simulink model "autonomous_vehicle"  (R2026a)
settings: Solver=VariableStepAuto  StopTime=2
values from neighbouring files (symbols this model uses):
  b = 2e-5    (= 2e-05)    [init_parameters.m]
  J = 2e-5    (= 2e-05)    [init_parameters.m]
  Ke = 0.02    [init_parameters.m]
  Kt = 0.02    [init_parameters.m]
  Ktheta = 2.0    (= 2)    [init_parameters.m]
  Ky = 1.0    (= 1)    [init_parameters.m]
  L = 2e-3    (= 0.002)    [init_parameters.m]
  R = 4    [init_parameters.m]
  theta0 = 0    [init_parameters.m]
  Vbase = 3.5    [init_parameters.m]
  Vmax = 6    [init_parameters.m]
  wheelDistance = 0.14    [init_parameters.m]
  wheelRadius = 0.0325    [init_parameters.m]
  x0 = 0    [init_parameters.m]
  y0 = 0.10    (= 0.1)    [init_parameters.m]
settings Model: Creator=aliad  LastModifiedBy=aliad

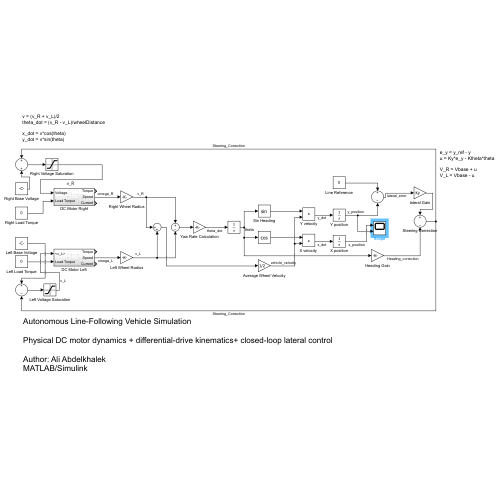
[thumbnail: Simulink's stored preview of the top-level diagram]
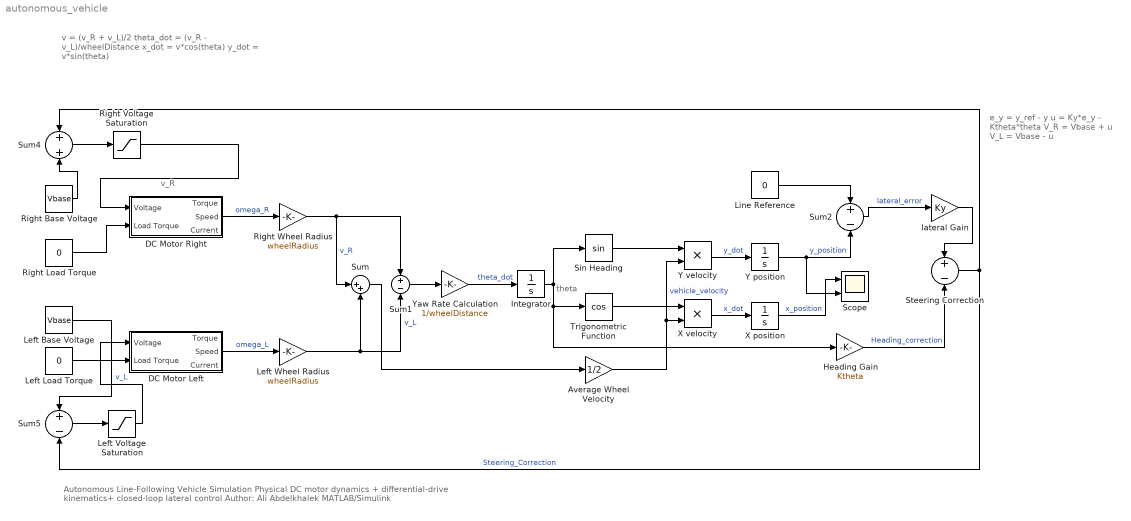
== system autonomous_vehicle ==
  note: v = (v_R + v_L)/2
      | theta_dot = (v_R - v_L)/wheelDistance
      |
      | x_dot = v*cos(theta)
      | y_dot = v*sin(theta)
  note: e_y = y_ref - y
      | u = Ky*e_y - Ktheta*theta
      |
      | V_R = Vbase + u
      | V_L = Vbase - u
  note: Autonomous Line-Following Vehicle Simulation
      |
      | Physical DC motor dynamics + differential-drive kinematics+ closed-loop lateral control
      |
      | Author: Ali Abdelkhalek
      | MATLAB/Simulink
  note: theta
  note: v_R
  "Average Wheel Velocity " : Gain  Gain=1/2
  DC Motor Left : Subsystem
  DC Motor Right : Subsystem
  Heading Gain : Gain  Gain=Ktheta
  Integrator : Integrator  InitialCondition=theta0
  Left Base Voltage : Constant  Value=Vbase
  Left Load Torque : Constant  Value=0
  Left Voltage Saturation : Saturate  UpperLimit=Vmax  LowerLimit=0
  Left Wheel Radius : Gain  Gain=wheelRadius
  Line Reference : Constant  Value=0
  Right Base Voltage : Constant  Value=Vbase
  Right Load Torque : Constant  Value=0
  Right Voltage Saturation : Saturate  UpperLimit=Vmax  LowerLimit=0
  Right Wheel Radius : Gain  Gain=wheelRadius
  Scope : Scope  NumInputPorts=2
      settings: ActiveDisplayYMinimum=-2.1385150832393238  ActiveDisplayYMaximum=5.3992745742207013
  Sin Heading : Trigonometry
  Steering Correction : Sum  Inputs=+-
  Sum : Sum  Inputs=|++
  Sum1 : Sum  Inputs=+-
  Sum2 : Sum  Inputs=+-
  Sum4 : Sum
  Sum5 : Sum  Inputs=+-
  Trigonometric Function : Trigonometry  Operator=cos
  X position : Integrator  InitialCondition=x0
  "X velocity " : Product
  Y position : Integrator  InitialCondition=y0
  Y velocity : Product
  Yaw Rate Calculation : Gain  Gain=1/wheelDistance
  lateral Gain : Gain  Gain=Ky
  wires:
  Left Load Torque/1 -> DC Motor Left/2(Load Torque)
  DC Motor Left/2(Speed) -> Left Wheel Radius/1  "omega_L"
  DC Motor Right/2(Speed) -> Right Wheel Radius/1  "omega_R"
  Right Load Torque/1 -> DC Motor Right/2(Load Torque)
  Sum/1 -> "Average Wheel Velocity "/1
  Left Wheel Radius/1 -> Sum1/2, Sum/2  "v_L"
  Right Wheel Radius/1 -> Sum1/1, Sum/1  "v_R"
  Sum1/1 -> Yaw Rate Calculation/1
  Yaw Rate Calculation/1 -> Integrator/1  "theta_dot"
  Integrator/1 -> Sin Heading/1, Heading Gain/1, Trigonometric Function/1
  Trigonometric Function/1 -> "X velocity "/1
  "Average Wheel Velocity "/1 -> Y velocity/2, "X velocity "/2  "vehicle_velocity"
  "X velocity "/1 -> X position/1  "x_dot"
  Sin Heading/1 -> Y velocity/1
  Y velocity/1 -> Y position/1  "y_dot"
  Y position/1 -> Scope/2, Sum2/2  "y_position"
  Line Reference/1 -> Sum2/1
  Sum2/1 -> lateral Gain/1  "lateral_error"
  lateral Gain/1 -> Steering Correction/1
  Heading Gain/1 -> Steering Correction/2  "Heading_correction"
  Steering Correction/1 -> Sum5/2, Sum4/1  "Steering_Correction"
  Right Base Voltage/1 -> Sum4/2
  Left Base Voltage/1 -> Sum5/1
  Sum4/1 -> Right Voltage Saturation/1
  Right Voltage Saturation/1 -> DC Motor Right/1(Voltage)
  Sum5/1 -> Left Voltage Saturation/1
  Left Voltage Saturation/1 -> DC Motor Left/1(Voltage)  "v_L"
  X position/1 -> Scope/1  "x_position"

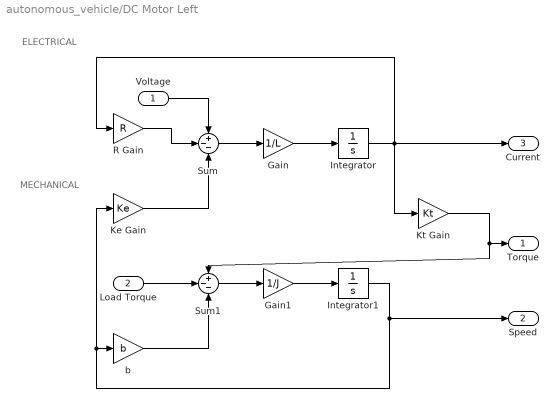
== system autonomous_vehicle/DC Motor Left ==
  note: ELECTRICAL
  note: MECHANICAL
  Voltage : Inport
  Load Torque : Inport  Port=2
  Gain : Gain  Gain=1/L
  Gain1 : Gain  Gain=1/J
  Integrator : Integrator
  Integrator1 : Integrator
  Ke Gain : Gain  Gain=Ke
  Kt Gain : Gain  Gain=Kt
  R Gain : Gain  Gain=R
  Sum : Sum  Inputs=+--
  Sum1 : Sum  Inputs=+--
  b : Gain  Gain=b
  " Torque" : Outport
  Speed : Outport  Port=2
  Current : Outport  Port=3
  wires:
  R Gain/1 -> Sum/2
  Integrator1/1 -> Speed/1, Ke Gain/1, b/1
  Kt Gain/1 -> " Torque"/1, Sum1/1
  Gain1/1 -> Integrator1/1
  Integrator/1 -> Kt Gain/1, Current/1, R Gain/1
  Load Torque/1 -> Sum1/2
  Gain/1 -> Integrator/1
  Ke Gain/1 -> Sum/3
  Sum/1 -> Gain/1
  Sum1/1 -> Gain1/1
  Voltage/1 -> Sum/1
  b/1 -> Sum1/3

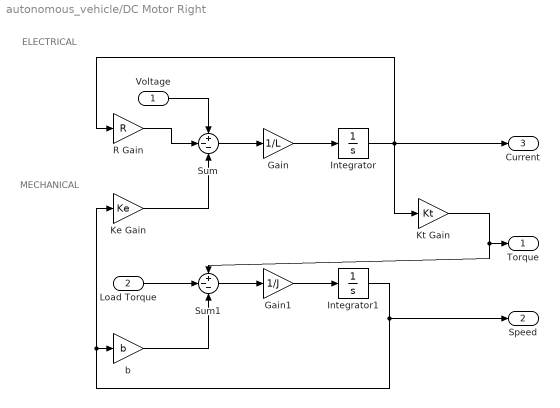
== system autonomous_vehicle/DC Motor Right ==
  note: ELECTRICAL
  note: MECHANICAL
  Voltage : Inport
  Load Torque : Inport  Port=2
  Gain : Gain  Gain=1/L
  Gain1 : Gain  Gain=1/J
  Integrator : Integrator
  Integrator1 : Integrator
  Ke Gain : Gain  Gain=Ke
  Kt Gain : Gain  Gain=Kt
  R Gain : Gain  Gain=R
  Sum : Sum  Inputs=+--
  Sum1 : Sum  Inputs=+--
  b : Gain  Gain=b
  " Torque" : Outport
  Speed : Outport  Port=2
  Current : Outport  Port=3
  wires:
  R Gain/1 -> Sum/2
  Integrator1/1 -> Speed/1, Ke Gain/1, b/1
  Kt Gain/1 -> " Torque"/1, Sum1/1
  Gain1/1 -> Integrator1/1
  Integrator/1 -> Kt Gain/1, Current/1, R Gain/1
  Load Torque/1 -> Sum1/2
  Gain/1 -> Integrator/1
  Ke Gain/1 -> Sum/3
  Sum/1 -> Gain/1
  Sum1/1 -> Gain1/1
  Voltage/1 -> Sum/1
  b/1 -> Sum1/3
